simulink model "Flow_Chart"  (R2021b)
settings: Solver=VariableStepAuto  StartTime=0.0  StopTime=10.0  RelTol=1e-3
undefined symbols (not defined in the file or in its folder): sigbuilder_block
settings Model: Creator=t  LastModifiedBy=t

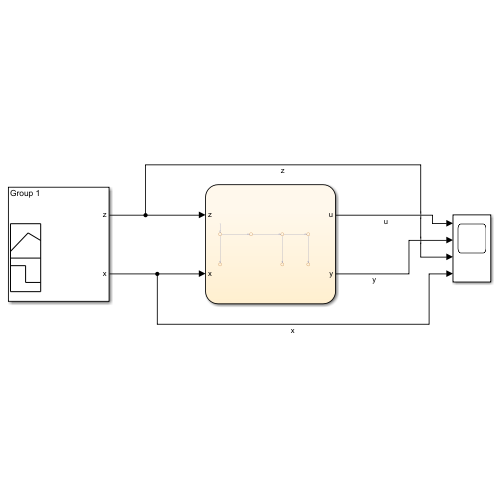
[thumbnail: Simulink's stored preview of the top-level diagram]
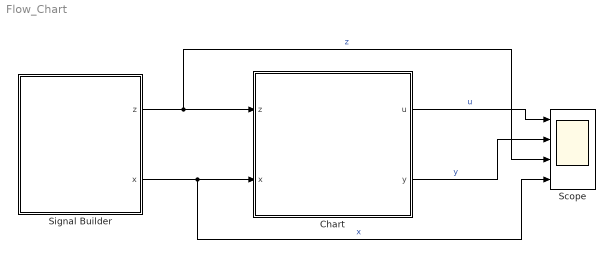
== system Flow_Chart ==
  Chart : Stateflow chart  TreatAsAtomicUnit=on
  Scope : Scope  NumInputPorts=4
  Signal Builder : Subsystem  Tag=STV Subsys  LoadFcn=sigbuilder_block('load');  StartFcn=sigbuilder_block('start');  StopFcn=sigbuilder_block('stop');  ClipboardFcn=sigbuilder_block('clipboard');  mask(Sigbuilder block){tuvar=[0:10]}
      mask help: Simulink:masks:SigbuilderBlock_MD
      mask init:
      | if ~strcmp(get_param(bdroot(gcbh),'SimulationStatus'),'stopped') tuvar = sigbuilder_block('maskInit'); end
      settings: CopyFcn=sigbuilder_block('copy');  DeleteFcn=sigbuilder_block('delete');  ModelCloseFcn=sigbuilder_block('modelClose');  PreSaveFcn=sigbuilder_block('preSave');  PauseFcn=sigbuilder_block('pause');  ContinueFcn=sigbuilder_block('continue');  NameChangeFcn=sigbuilder_block('namechange');  OpenFcn=sigbuilder_block('open',[134.4 63 550.8 400.2 ]);  CloseFcn=sigbuilder_block('close');
      mask Display: plot(0, 0, 100, 100,[2, 2, 32, 32, 2], [68, 8, 8, 68, 68],[32, 2], [38, 38], [32, 19, 2],[53, 60, 44], [32, 17, 17, 2],[16, 16, 31, 31]);txt = getActiveGroup(gcbh);text(2, 100, txt,'verticalAlignment', 'top');
  wires:
  Chart/1(u) -> Scope/1  "u"
  Chart/2(y) -> Scope/2  "y"
  Signal Builder/1(z) -> Scope/3, Chart/1(z)  "z"
  Signal Builder/2(x) -> Scope/4, Chart/2(x)  "x"

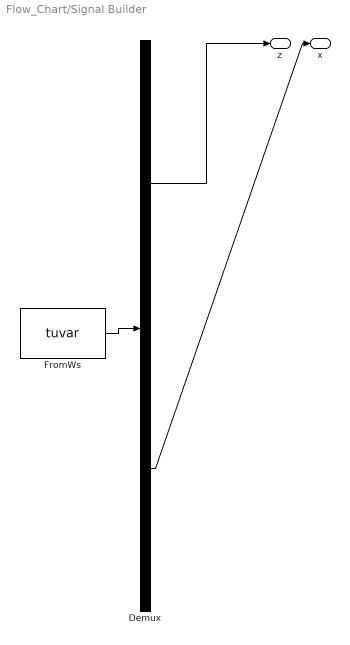
== system Flow_Chart/Signal Builder ==
  Demux : Demux  Tag=STV Demux  Outputs=2
      settings: DisplayOption=none
  FromWs : FromWorkspace  Tag=STV FromWs  VariableName=tuvar
      SigBuilderData=|
      | common.afterFinalStr = 'Extrapolate'
      | common.sampleTime = 0
      | dataSet.timeRange = [0 10]
      | dataSet.name = 'Group 1'
      | sbobj.Groups.Name = 'Group 1'
      | sbobj.Groups.Signals(1).Name = 'z'
      | sbobj.Groups.Signals(1).XData = [0 2 2 4 4 6 6 7.7 7.7 9.16 9.16 10]
      | sbobj.Groups.Signals(1).YData = [5 5 4 4 5 5 0 0 5 5 2 2]
      | sbobj.Groups.Signals(2).Name = 'x'
      | sbobj.Groups.Signals(2).XData = [0 7 7 10]
      | sbobj.Groups.Signals(2).YData = [0 0 0.54 0.54]
  z : Outport  Tag=STV Outport
  x : Outport  Tag=STV Outport  Port=2
  wires:
  Demux/1 -> z/1
  FromWs/1 -> Demux/1
  Demux/2 -> x/1

== stateflow chart Flow_Chart/Chart ==
  (default) -> (junction 1)
  (junction 1) -> (junction 3) [order 1] : [x==0]
  (junction 3) -> (junction 4) : {y=1;}
  (junction 4) -> (junction 5) [order 1] : [z==5]
  (junction 1) -> (junction 9) [order 2] : {y=2;}
  (junction 4) -> (junction 6) [order 2] : {u=20;}
  (junction 5) -> (junction 7) : {u=15;}
  data: z input; x input; u output; y output
